simulink model "phase_opt"  (R2017b)
settings: Solver=FixedStepDiscrete  StartTime=0.0  StopTime=2e-3  FixedStep=1/162.5e6  RelTol=1e-3
libraries: Library_SignalGeneration x8
settings Model: Creator=sawmilkd  LastModifiedBy=sawmilkd

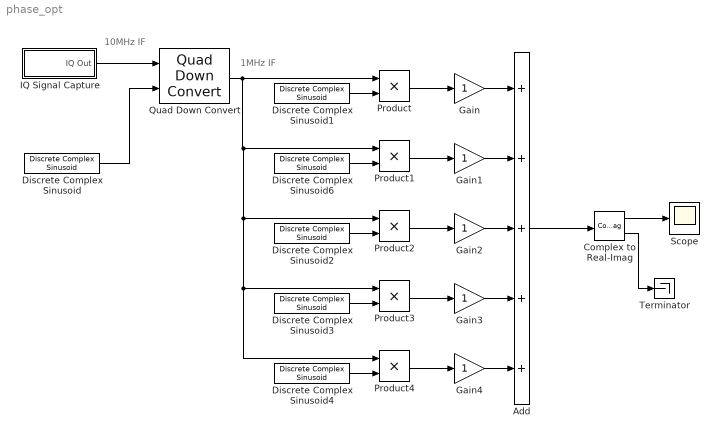
== system phase_opt ==
  note: 1MHz IF
  note: 10MHz IF
  Add : Sum  Inputs=+++++
  Complex to Real-Imag : ComplexToRealImag
  Discrete Complex Sinusoid : Library_SignalGeneration/Discrete Complex Sinusoid  initPhase=0  freqHz=9e6
      settings: AttributesFormatString=Frequency: %<freqHz>
  Discrete Complex Sinusoid1 : Library_SignalGeneration/Discrete Complex Sinusoid  initPhase=pi  freqHz=1e6-2000
      settings: AttributesFormatString=|
      | Frequency: %<freqHz>
      | Starting Phase: %<initPhase>
  Discrete Complex Sinusoid2 : Library_SignalGeneration/Discrete Complex Sinusoid  initPhase=0*pi/180  freqHz=1e6
      settings: AttributesFormatString=|
      | Frequency: %<freqHz>
      | Starting Phase: %<initPhase>
  Discrete Complex Sinusoid3 : Library_SignalGeneration/Discrete Complex Sinusoid  initPhase=0  freqHz=1e6+1000.
      settings: AttributesFormatString=|
      | Frequency: %<freqHz>
      | Starting Phase: %<initPhase>
  Discrete Complex Sinusoid4 : Library_SignalGeneration/Discrete Complex Sinusoid  initPhase=pi/2  freqHz=1e6+2000
      settings: AttributesFormatString=|
      | Frequency: %<freqHz>
      | Starting Phase: %<initPhase>
  Discrete Complex Sinusoid6 : Library_SignalGeneration/Discrete Complex Sinusoid  initPhase=pi/4  freqHz=1e6-1000
      settings: AttributesFormatString=|
      | Frequency: %<freqHz>
      | Starting Phase: %<initPhase>
  Gain{,1..4} (5 alike) : Gain
  IQ Signal Capture : Subsystem
  Product{,1..4} (5 alike) : Product
  Quad Down Convert : Library_SignalGeneration/Quad Down Convert  SystemSampleTime=-1
  Scope : Scope
  Terminator : Terminator
  wires:
  IQ Signal Capture/1(IQ Out) -> Quad Down Convert/1
  Discrete Complex Sinusoid/1 -> Quad Down Convert/2
  Quad Down Convert/1 -> Product3/1, Product4/1, Product2/1, Product1/1, Product/1
  Discrete Complex Sinusoid1/1 -> Product/2
  Discrete Complex Sinusoid6/1 -> Product1/2
  Discrete Complex Sinusoid2/1 -> Product2/2
  Discrete Complex Sinusoid3/1 -> Product3/2
  Discrete Complex Sinusoid4/1 -> Product4/2
  Product/1 -> Gain/1
  Product4/1 -> Gain4/1
  Product3/1 -> Gain3/1
  Product2/1 -> Gain2/1
  Product1/1 -> Gain1/1
  Gain2/1 -> Add/3
  Gain1/1 -> Add/2
  Gain/1 -> Add/1
  Gain3/1 -> Add/4
  Gain4/1 -> Add/5
  Add/1 -> Complex to Real-Imag/1
  Complex to Real-Imag/1 -> Scope/1
  Complex to Real-Imag/2 -> Terminator/1

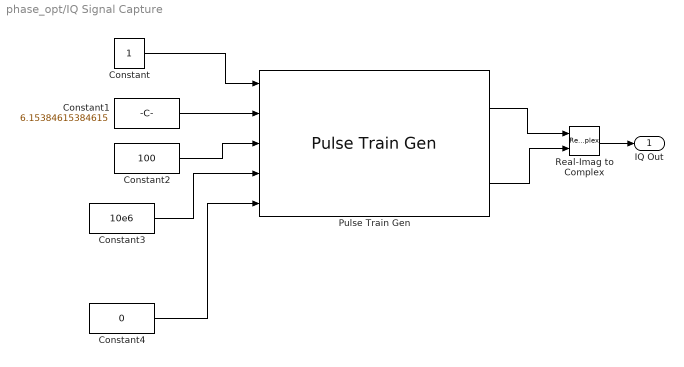
== system phase_opt/IQ Signal Capture ==
  Constant : Constant
  Constant1 : Constant  Value=6.15384615384615
  Constant2 : Constant  Value=100
  Constant3 : Constant  Value=10e6
  Constant4 : Constant  Value=0
  Pulse Train Gen : Library_SignalGeneration/Pulse Train Gen
  Real-Imag to Complex : RealImagToComplex
  IQ Out : Outport
  wires:
  Constant/1 -> Pulse Train Gen/1
  Constant1/1 -> Pulse Train Gen/2
  Constant3/1 -> Pulse Train Gen/4
  Constant4/1 -> Pulse Train Gen/5
  Constant2/1 -> Pulse Train Gen/3
  Pulse Train Gen/1 -> Real-Imag to Complex/1
  Pulse Train Gen/2 -> Real-Imag to Complex/2
  Real-Imag to Complex/1 -> IQ Out/1
